simulink model "lr_pwm"  (R2021b)
settings: Solver=ode1  StartTime=0.0  StopTime=3  FixedStep=T_sim  RelTol=1e-3  AbsTol=1e-3
values from neighbouring files (symbols this model uses):
  Ac_s = [-1/(C_s*R_s)    1/C_s ... (first row only)    [lr_pwm_data.m]
  Ao_s = [-1/(C_s*R_s)    1/C_s ... (first row only)    [lr_pwm_data.m]
  Bc_s = [0;1/L_l]    [lr_pwm_data.m]
  Bo_s = [0;1/(L_l)]    [lr_pwm_data.m]
  Cc_s = [1/R_s 0]    [lr_pwm_data.m]
  Co_s = [0 1]    [lr_pwm_data.m]
  Dc_s = zeros(p,m)    [lr_pwm_data.m]
  delta = 0.001    [lr_pwm_data.m]
  deltao = 0.001    [lr_pwm_data.m]
  FR = -diag([1/0.01])    [lr_pwm_data.m]
  L = 200e-3    (= 0.2)    [Parameter_Vergleich.m]
  Lam_inv = inv(Lam)    [lr_pwm_data.m]
  R_l = 4    [lr_pwm_data.m]
  R_s = 0.1    [lr_pwm_data.m]
  rho = 1    [lr_pwm_data.m]
  rhoo = 5    [lr_pwm_data.m]
  SampleTime = 0.001    [lr_pwm_data.m]
  To_inv = eye(n)    [lr_pwm_data.m]
  U_e = 12    [Parameter_Vergleich.m]    (also in lr_pwm_data.m = 12.5)
  xb0_z = ( eye(length(Ab_z)) - Ab_z ) \ Bb_z * u0    [lr_pwm_data.m]
  xc0_s = ( -Ac_s ) * Bc_s .\ u0    [lr_pwm_data.m]
  xc0_z = ( eye(length(Ac_z)) - Ac_z ) \ Bc_z * u0    [lr_pwm_data.m]
  z0 = zeros(1,n)    [lr_pwm_data.m]
undefined symbols (not defined in the file or in its folder): Ab_z, Ac_z, Bb_z, Bc_z, Cb_z, Cc_z, Db_z, Dc_z, DiscIntNeverNeededParam, F, G, Lr, Lrdot, P, S, Sr
libraries: fl_lib x22, nesl_utility x12, simulink x5, ee_lib x1
Description:
  | PWM-Controlled DC Motor
settings Model: DataTypeOverride=Off  MinMaxOverflowLogging=ForceOff  SimulationMode=accelerator  Creator=The MathWorks, Inc.  LastModifiedBy=w.schwamm
settings SolverCC: AutoScaleAbsTol=off  AlgebraicLoopSolver=TrustRegion
settings DataIOCC: LimitDataPoints=on  MaxDataPoints=10000  SaveOutput=off  SaveTime=off  SignalLoggingName=logsout_lr_pwm
settings OptimizationCC: DefaultParameterBehavior=Inlined  EnhancedBackFolding=on  PassReuseOutputArgsAs=Individual arguments  ExpressionDepthLimit=2147483647  ZeroExternalMemoryAtStartup=off  ZeroInternalMemoryAtStartup=off  InitFltsAndDblsToZero=on  OptimizeBlockOrder=speed  DifferentSizesBufferReuse=on  OptimizationCustomize=off  EfficientTunableParamExpr=on
settings DebuggingCC: SignalRangeChecking=error  UnderspecifiedInitializationDetection=Classic  MergeDetectMultiDrivingBlocksExec=none  IntegerOverflowMsg=none  ParameterDowncastMsg=none  ParameterOverflowMsg=none  ParameterPrecisionLossMsg=none  ParameterTunabilityLossMsg=error  FcnCallInpInsideContextMsg=warning  StateNameClashWarn=warning  SFUnexpectedBacktrackingDiag=warning  SFNoUnconditionalDefaultTransitionDiag=warning  SFExecutionAtInitializationDiag=none  SFMachineParentedDataDiag=warning  IntegerSaturationMsg=none  ArithmeticOperatorsInVariantConditions=warning
settings HardwareCC: ProdBitPerPointer=32  ProdBitPerSizeT=32  ProdBitPerPtrDiffT=32  ProdLargestAtomicInteger=Long  ProdLargestAtomicFloat=Double  ProdWordSize=32  ProdHWDeviceType=ARM Compatible->ARM 11
settings ModelReferenceCC: PropagateSignalLabelsOutOfModel=off
settings SFSimCC: SimUseLocalCustomCode=off  MATLABDynamicMemAlloc=off  CustomCodeUndefinedFunction=UseInterfaceOnly
settings RTWCC: Description=Embedded Coder  SystemTargetFile=ert.tlc  TemplateMakefile=ert_default_tmf  RTWUseLocalCustomCode=off
settings CodeAppCC: ForceParamTrailComments=on  IgnoreCustomStorageClasses=off  OperatorAnnotations=on  SimulinkDataObjDesc=on  SFDataObjDesc=on  InsertBlockDesc=on
settings ERTTargetCC: GenerateSampleERTMain=on  InlinedParameterPlacement=NonHierarchical  ERTCustomFileTemplate=example_file_process.tlc
settings ConfigComp: CovMetricSettings=dw  CovSaveCumulativeToWorkspaceVar=on  CovSaveSingleToWorkspaceVar=on  CovExternalEMLEnable=off  CovSFcnEnable=off
settings SimscapeCC: SimscapeLogType=all  SimscapeLogSimulationStatistics=on  SimscapeLogName=simlog_lr_pwm  SimscapeLogDataHistory=10000

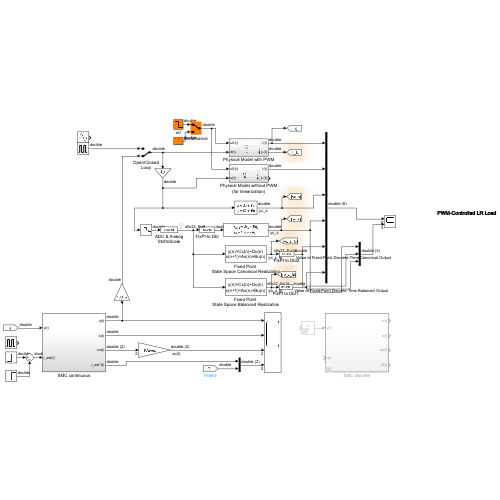
[thumbnail: Simulink's stored preview of the top-level diagram]
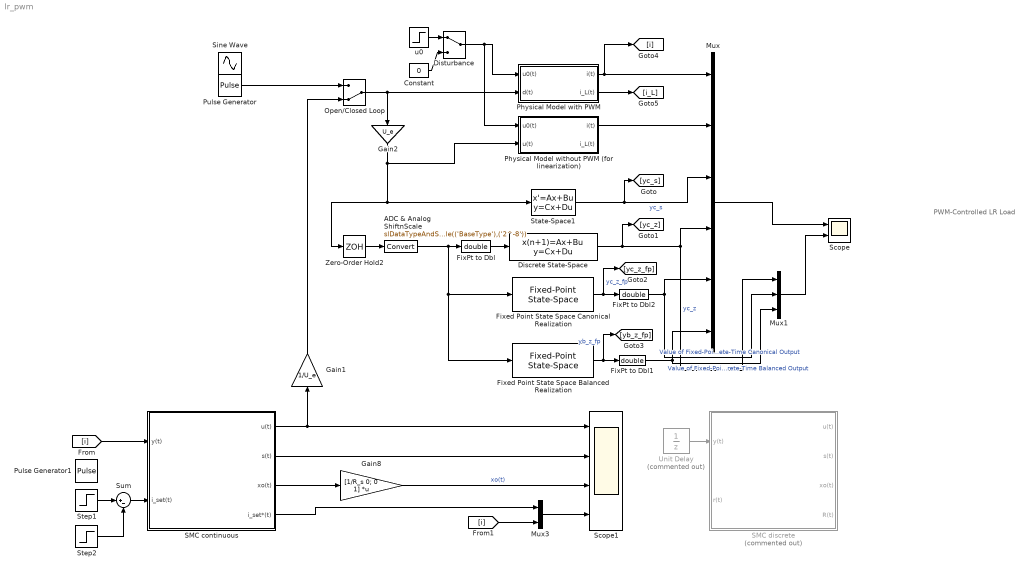
== system lr_pwm ==
  note: PWM-Controlled LR Load
  ADC & Analog ShiftnScale : DataTypeConversion  OutDataTypeStr=slDataTypeAndScale(('BaseType'),('2^-8'))  RndMeth=Nearest  SaturateOnIntegerOverflow=on  LockScale=on
  Constant : Constant  Value=0
  Discrete State-Space : DiscreteStateSpace  A=Ac_z  B=Bc_z  C=Cc_z  D=Dc_z  InitialCondition=xc0_z  SampleTime=SampleTime
  Disturbance : ManualSwitch
  FixPt to Dbl : DataTypeConversion  OutDataTypeStr=double
  FixPt to Dbl1 : DataTypeConversion  OutDataTypeStr=double
  FixPt to Dbl2 : DataTypeConversion  OutDataTypeStr=double
  Fixed Point State Space Balanced Realization : simulink/Additional Math & Discrete/Additional Discrete/Fixed-Point State-Space  A=Ab_z  B=Bb_z  C=Cb_z  D=Db_z  InitialCondition=xb0_z  InternalDataType=BaseType  StateEqScaling=2^(-13)  OutputEqScaling=2^(-15)  DoSatur=off
      settings: SourceProductBaseCode=SL
  Fixed Point State Space Canonical Realization : simulink/Additional Math & Discrete/Additional Discrete/Fixed-Point State-Space  A=Ac_z  B=Bc_z  C=Cc_z  D=Dc_z  InitialCondition=xc0_z  InternalDataType=BaseType  StateEqScaling=2^(-13)  OutputEqScaling=2^(-15)  DoSatur=off
      settings: SourceProductBaseCode=SL
  Gain1 : Gain  Gain=1/U_e
  Gain2 : Gain  Gain=U_e
  Gain8 : Gain  Gain=[1/R_s 0; 0 1]  Multiplication=Matrix(K*u) (u vector)
  Mux : Mux  Inputs=6
  Mux1 : Mux  Inputs=3
  Mux3 : Mux  Inputs=2
  Open/Closed Loop : ManualSwitch  CurrentSetting=0
  Physical Model with PWM : Subsystem
  Physical Model without PWM (for linearization) : Subsystem
  Pulse Generator : DiscretePulseGenerator  PulseType=Time based  Period=0.5  PulseWidth=50
  Pulse Generator1 : DiscretePulseGenerator  PulseType=Time based  Amplitude=1.5  Period=0.5  PulseWidth=50
  SMC continuous : Subsystem  SystemSampleTime=0.001
  SMC discrete : Subsystem  Commented=on  TreatAsAtomicUnit=on  SystemSampleTime=0.001
  Scope : Scope  NumInputPorts=2
  Scope1 : Scope  NumInputPorts=4
  Sine Wave : Sin  Amplitude=0.5  Bias=0.5  Frequency=50  SampleTime=0
  State-Space1 : StateSpace  A=Ac_s  B=Bc_s  C=Cc_s  D=Dc_s  InitialCondition=xc0_s
  Step1 : Step  Time=0.1  After=1.0  SampleTime=0
  Step2 : Step  Time=2  After=0.5  SampleTime=0
  Sum : Sum  Inputs=|+-
  Unit Delay : UnitDelay  Commented=on  SampleTime=-1  HasFrameUpgradeWarning=on
  Zero-Order Hold2 : ZeroOrderHold  SampleTime=SampleTime
  u0 : Step  Time=0.5  After=-3  SampleTime=0
  wires:
  Mux/1 -> Scope/1
  Physical Model without PWM (for linearization)/1(i(t)) -> Mux/2
  State-Space1/1 -> [yc_s], Mux/3  "yc_s"
  Zero-Order Hold2/1 -> ADC & Analog ShiftnScale/1
  ADC & Analog ShiftnScale/1 -> Fixed Point State Space Balanced Realization/1, Fixed Point State Space Canonical Realization/1, FixPt to Dbl/1
  FixPt to Dbl/1 -> Discrete State-Space/1
  Discrete State-Space/1 -> [yc_z], Mux/4, Mux1/1  "yc_z"
  Fixed Point State Space Canonical Realization/1 -> [yc_z_fp], FixPt to Dbl2/1  "yc_z_fp"
  Fixed Point State Space Balanced Realization/1 -> [yb_z_fp], FixPt to Dbl1/1  "yb_z_fp"
  Physical Model with PWM/1(i(t)) -> [i], Mux/1
  FixPt to Dbl2/1 -> Mux1/2, Mux/5  "Value of Fixed-Point Discrete-Time Canonical Output"
  Mux1/1 -> Scope/2
  FixPt to Dbl1/1 -> Mux/6, Mux1/3  "Value of Fixed-Point Discrete-Time Balanced Output"
  Physical Model with PWM/2(i_L(t)) -> [i_L]
  [i] -> Mux3/2
  SMC continuous/1(u(t)) -> Scope1/1, Gain1/1
  Mux3/1 -> Scope1/4
  SMC continuous/2(s(t)) -> Scope1/2
  SMC continuous/3(xo(t)) -> Gain8/1
  Gain8/1 -> Scope1/3  "xo(t)"
  SMC continuous/4(i_set*(t)) -> Mux3/1
  Gain1/1 -> Open/Closed Loop/2
  Step1/1 -> Sum/1
  Sum/1 -> SMC continuous/2(i_set(t))
  Step2/1 -> Sum/2
  u0/1 -> Disturbance/1
  Constant/1 -> Disturbance/2
  Disturbance/1 -> Physical Model without PWM (for linearization)/1(u0(t)), Physical Model with PWM/1(u0(t))
  Open/Closed Loop/1 -> Gain2/1, Physical Model with PWM/2(d(t))
  Pulse Generator/1 -> Open/Closed Loop/1
  Gain2/1 -> Physical Model without PWM (for linearization)/2(u(t)), Zero-Order Hold2/1, State-Space1/1
  Unit Delay/1 -> SMC discrete/1(y(t))
  [i] -> SMC continuous/1(y(t))

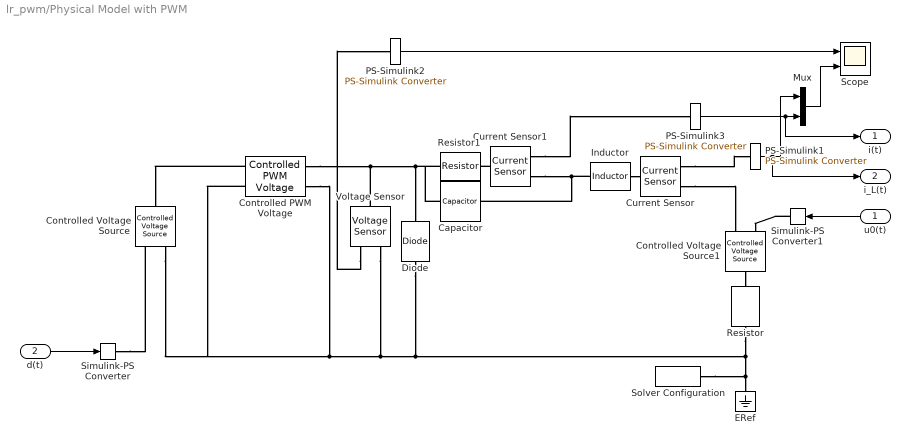
== system lr_pwm/Physical Model with PWM ==
  u0(t) : Inport
  d(t) : Inport  Port=2
  Capacitor : fl_lib/Electrical/Electrical Elements/Capacitor  c=C_s F  r=0 Ohm  g=0 1/Ohm  i_specify=off  i_priority=None  i=0 A  i_nominal_specify=off  i_nominal_unit=A  i_nominal_value=1  v_specify=off  v_priority=None  v=0 V  v_nominal_specify=off  v_nominal_unit=V  v_nominal_value=1  vc_specify=off  vc_priority=High  vc=0 V  vc_nominal_specify=off  vc_nominal_unit=V  vc_nominal_value=1
  Controlled PWM Voltage : ee_lib/Integrated Circuits/Controlled PWM Voltage  F=f_pwm Hz  TD=0 s  pulse_width_offset=0 s  pulse_min=0 s  pwm_or_av=1  event_type=2  sample_time=T_sim s  Vmin=0 V  Vmax=1 V  Vm=U_e V  u_min=0  u_max=1
  Controlled Voltage Source : fl_lib/Electrical/Electrical Sources/Controlled Voltage Source
  Controlled Voltage Source1 : fl_lib/Electrical/Electrical Sources/Controlled Voltage Source
  Current Sensor : fl_lib/Electrical/Electrical Sensors/Current Sensor
  Current Sensor1 : fl_lib/Electrical/Electrical Sensors/Current Sensor
  Diode : fl_lib/Electrical/Electrical Elements/Diode  Vf=0.6 V  Ron=0.3 Ohm  Goff=1e-8 1/Ohm  i_specify=off  i_priority=None  i=0 A  i_nominal_specify=off  i_nominal_unit=A  i_nominal_value=1  v_specify=off  v_priority=None  v=0 V  v_nominal_specify=off  v_nominal_unit=V  v_nominal_value=1
  ERef : fl_lib/Electrical/Electrical Elements/Electrical Reference
  Inductor : fl_lib/Electrical/Electrical Elements/Inductor  l=L_l H  r=0 Ohm  g=0 1/Ohm  i_specify=off  i_priority=None  i=0 A  i_nominal_specify=off  i_nominal_unit=A  i_nominal_value=1  v_specify=off  v_priority=None  v=0 V  v_nominal_specify=off  v_nominal_unit=V  v_nominal_value=1  i_L_specify=off  i_L_priority=High  i_L=0 A  i_L_nominal_specify=off  i_L_nominal_unit=A  i_L_nominal_value=1
  Mux : Mux  Inputs=2
  PS-Simulink1 : nesl_utility/PS-Simulink Converter  PhysicalDomain=network_engine_domain  SubClassName=ps_output  LeftPortType=input  RightPortType=output  PseudoPeriodic=off  Frequencies=[]  Unit=A  AffineConversion=off
      settings: SourceProductBaseCode=PW,SS
  PS-Simulink2 : nesl_utility/PS-Simulink Converter  PhysicalDomain=network_engine_domain  SubClassName=ps_output  LeftPortType=input  RightPortType=output  PseudoPeriodic=off  Frequencies=[]  Unit=V  AffineConversion=off
      settings: SourceProductBaseCode=PW,SS
  PS-Simulink3 : nesl_utility/PS-Simulink Converter  PhysicalDomain=network_engine_domain  SubClassName=ps_output  LeftPortType=input  RightPortType=output  PseudoPeriodic=off  Frequencies=[]  Unit=A  AffineConversion=off
      settings: SourceProductBaseCode=PW,SS
  Resistor : fl_lib/Electrical/Electrical Elements/Resistor  R=R_l Ohm  i_specify=off  i_priority=None  i=0 A  i_nominal_specify=off  i_nominal_unit=A  i_nominal_value=1  v_specify=off  v_priority=None  v=0 V  v_nominal_specify=off  v_nominal_unit=V  v_nominal_value=1
  Resistor1 : fl_lib/Electrical/Electrical Elements/Resistor  R=R_s Ohm  i_specify=off  i_priority=None  i=0 A  i_nominal_specify=off  i_nominal_unit=A  i_nominal_value=1  v_specify=off  v_priority=None  v=0 V  v_nominal_specify=off  v_nominal_unit=V  v_nominal_value=1
  Scope : Scope  NumInputPorts=2
  Simulink-PS Converter : nesl_utility/Simulink-PS Converter  PhysicalDomain=network_engine_domain  SubClassName=ps_input  LeftPortType=input  RightPortType=output  PseudoPeriodic=off  Frequencies=[]  NoiseDistribution=none  NoiseParameters=[]  Unit=1  AffineConversion=off  FilteringAndDerivatives=filter  SimscapeFilterOrder=1  InputFilterTimeConstant=0.001  UdotUserProvided=0
      settings: SourceProductBaseCode=PW,SS
  Simulink-PS Converter1 : nesl_utility/Simulink-PS Converter  PhysicalDomain=network_engine_domain  SubClassName=ps_input  LeftPortType=input  RightPortType=output  PseudoPeriodic=off  Frequencies=[]  NoiseDistribution=none  NoiseParameters=[]  Unit=V  AffineConversion=off  FilteringAndDerivatives=filter  SimscapeFilterOrder=1  InputFilterTimeConstant=0.001  UdotUserProvided=0
      settings: SourceProductBaseCode=PW,SS
  Solver Configuration : nesl_utility/Solver Configuration  PhysicalDomain=network_engine_domain  SubClassName=solver  LeftPortType=input  RightPortType=generic  Tones=[]  Harmonics=[]  SimulateNoise=off  Profile=off  UseLocalSampling=off  EnableSwitchedLinearOptims=on  FrequencyDomain=off  UseCCode=off  RelTol=0.001  AbsTol=1e-06  MinStep=1e-09  ToWorkspace=off  RevertToSquareIcSolve=off  NumHomotopyIterations=100  PhasorMode=off  PhasorModeNumHarmonics=1  DoDC=off  ResidualTolerance=1e-9  UseLocalSolver=off  LocalSolverChoice=NE_BACKWARD_EULER_ADVANCER  LocalSolverSampleTime=5e-6  DoFixedCost=off  MaxNonlinIter=4  MaxModeIter=2  ComputeImpulses=off  ImpulseIterations=2  LinearAlgebra=auto  EquationFormulation=NE_TIME_EF  DelaysMemoryBudget=1024  AutomaticFiltering=off  FilteringTimeConstant=0.001  PartitionStorageMethod=AS_NEEDED  PartitionMemoryBudget=1024  PartitionMethod=FAST
      settings: SourceProductBaseCode=PW,SS
  Voltage Sensor : fl_lib/Electrical/Electrical Sensors/Voltage Sensor
  i(t) : Outport
  i_L(t) : Outport  Port=2
  wires:
  PS-Simulink2/1 -> Scope/1
  d(t)/1 -> Simulink-PS Converter/1
  PS-Simulink3/1 -> i(t)/1, Mux/2
  Mux/1 -> Scope/2
  PS-Simulink1/1 -> i_L(t)/1, Mux/1
  u0(t)/1 -> Simulink-PS Converter1/1
  connections:
  Voltage Sensor/LConn1 -- Capacitor/LConn1 -- Resistor1/LConn1 -- Diode/RConn1 -- Controlled PWM Voltage/RConn1
  Inductor/RConn1 -- Current Sensor/LConn1
  Voltage Sensor/RConn2 -- Controlled PWM Voltage/RConn2 -- Controlled PWM Voltage/LConn2 -- Controlled Voltage Source/RConn2 -- Diode/LConn1 -- Resistor/RConn1 -- Solver Configuration/RConn1 -- ERef/LConn1
  Inductor/LConn1 -- Current Sensor1/RConn2 -- Capacitor/RConn1
  Simulink-PS Converter/RConn1 -- Controlled Voltage Source/RConn1
  Current Sensor1/LConn1 -- Resistor1/RConn1
  Current Sensor1/RConn1 -- PS-Simulink3/LConn1
  Current Sensor/RConn1 -- PS-Simulink1/LConn1
  Voltage Sensor/RConn1 -- PS-Simulink2/LConn1
  Controlled PWM Voltage/LConn1 -- Controlled Voltage Source/LConn1
  Simulink-PS Converter1/RConn1 -- Controlled Voltage Source1/RConn1
  Controlled Voltage Source1/LConn1 -- Resistor/LConn1
  Current Sensor/RConn2 -- Controlled Voltage Source1/RConn2

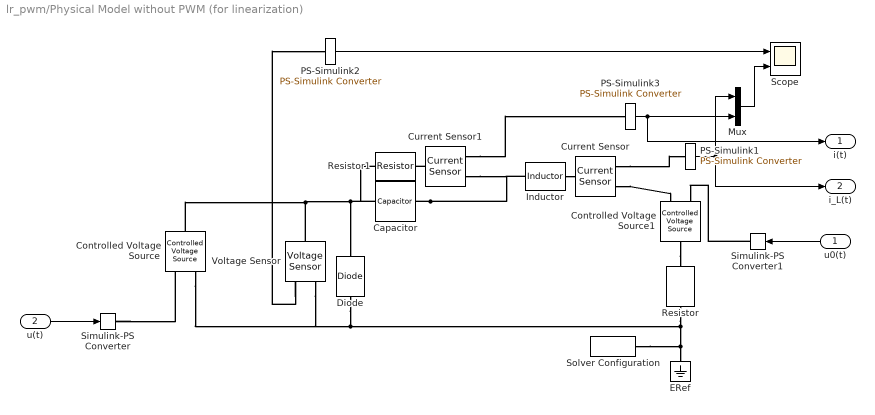
== system lr_pwm/Physical Model without PWM (for linearization) ==
  u0(t) : Inport
  u(t) : Inport  Port=2
  Capacitor : fl_lib/Electrical/Electrical Elements/Capacitor  c=C_s F  r=0 Ohm  g=0 1/Ohm  i_specify=off  i_priority=None  i=0 A  i_nominal_specify=off  i_nominal_unit=A  i_nominal_value=1  v_specify=off  v_priority=None  v=0 V  v_nominal_specify=off  v_nominal_unit=V  v_nominal_value=1  vc_specify=off  vc_priority=High  vc=0 V  vc_nominal_specify=off  vc_nominal_unit=V  vc_nominal_value=1
  Controlled Voltage Source : fl_lib/Electrical/Electrical Sources/Controlled Voltage Source
  Controlled Voltage Source1 : fl_lib/Electrical/Electrical Sources/Controlled Voltage Source
  Current Sensor : fl_lib/Electrical/Electrical Sensors/Current Sensor
  Current Sensor1 : fl_lib/Electrical/Electrical Sensors/Current Sensor
  Diode : fl_lib/Electrical/Electrical Elements/Diode  Vf=0.6 V  Ron=0.3 Ohm  Goff=1e-8 1/Ohm  i_specify=off  i_priority=None  i=0 A  i_nominal_specify=off  i_nominal_unit=A  i_nominal_value=1  v_specify=off  v_priority=None  v=0 V  v_nominal_specify=off  v_nominal_unit=V  v_nominal_value=1
  ERef : fl_lib/Electrical/Electrical Elements/Electrical Reference
  Inductor : fl_lib/Electrical/Electrical Elements/Inductor  l=L_l H  r=0 Ohm  g=0 1/Ohm  i_specify=off  i_priority=None  i=0 A  i_nominal_specify=off  i_nominal_unit=A  i_nominal_value=1  v_specify=off  v_priority=None  v=0 V  v_nominal_specify=off  v_nominal_unit=V  v_nominal_value=1  i_L_specify=off  i_L_priority=High  i_L=0 A  i_L_nominal_specify=off  i_L_nominal_unit=A  i_L_nominal_value=1
  Mux : Mux  Inputs=2
  PS-Simulink1 : nesl_utility/PS-Simulink Converter  PhysicalDomain=network_engine_domain  SubClassName=ps_output  LeftPortType=input  RightPortType=output  PseudoPeriodic=off  Frequencies=[]  Unit=A  AffineConversion=off
      settings: SourceProductBaseCode=PW,SS
  PS-Simulink2 : nesl_utility/PS-Simulink Converter  PhysicalDomain=network_engine_domain  SubClassName=ps_output  LeftPortType=input  RightPortType=output  PseudoPeriodic=off  Frequencies=[]  Unit=V  AffineConversion=off
      settings: SourceProductBaseCode=PW,SS
  PS-Simulink3 : nesl_utility/PS-Simulink Converter  PhysicalDomain=network_engine_domain  SubClassName=ps_output  LeftPortType=input  RightPortType=output  PseudoPeriodic=off  Frequencies=[]  Unit=A  AffineConversion=off
      settings: SourceProductBaseCode=PW,SS
  Resistor : fl_lib/Electrical/Electrical Elements/Resistor  R=R_l Ohm  i_specify=off  i_priority=None  i=0 A  i_nominal_specify=off  i_nominal_unit=A  i_nominal_value=1  v_specify=off  v_priority=None  v=0 V  v_nominal_specify=off  v_nominal_unit=V  v_nominal_value=1
  Resistor1 : fl_lib/Electrical/Electrical Elements/Resistor  R=R_s Ohm  i_specify=off  i_priority=None  i=0 A  i_nominal_specify=off  i_nominal_unit=A  i_nominal_value=1  v_specify=off  v_priority=None  v=0 V  v_nominal_specify=off  v_nominal_unit=V  v_nominal_value=1
  Scope : Scope  NumInputPorts=2
  Simulink-PS Converter : nesl_utility/Simulink-PS Converter  PhysicalDomain=network_engine_domain  SubClassName=ps_input  LeftPortType=input  RightPortType=output  PseudoPeriodic=off  Frequencies=[]  NoiseDistribution=none  NoiseParameters=[]  Unit=1  AffineConversion=off  FilteringAndDerivatives=provide  SimscapeFilterOrder=1  InputFilterTimeConstant=0.001  UdotUserProvided=0
      settings: SourceProductBaseCode=PW,SS
  Simulink-PS Converter1 : nesl_utility/Simulink-PS Converter  PhysicalDomain=network_engine_domain  SubClassName=ps_input  LeftPortType=input  RightPortType=output  PseudoPeriodic=off  Frequencies=[]  NoiseDistribution=none  NoiseParameters=[]  Unit=V  AffineConversion=off  FilteringAndDerivatives=filter  SimscapeFilterOrder=1  InputFilterTimeConstant=0.001  UdotUserProvided=0
      settings: SourceProductBaseCode=PW,SS
  Solver Configuration : nesl_utility/Solver Configuration  PhysicalDomain=network_engine_domain  SubClassName=solver  LeftPortType=input  RightPortType=generic  Tones=[]  Harmonics=[]  SimulateNoise=off  Profile=off  UseLocalSampling=off  EnableSwitchedLinearOptims=on  FrequencyDomain=off  UseCCode=off  RelTol=0.001  AbsTol=1e-06  MinStep=1e-09  ToWorkspace=off  RevertToSquareIcSolve=off  NumHomotopyIterations=100  PhasorMode=off  PhasorModeNumHarmonics=1  DoDC=off  ResidualTolerance=1e-9  UseLocalSolver=off  LocalSolverChoice=NE_BACKWARD_EULER_ADVANCER  LocalSolverSampleTime=5e-6  DoFixedCost=off  MaxNonlinIter=4  MaxModeIter=2  ComputeImpulses=off  ImpulseIterations=2  LinearAlgebra=auto  EquationFormulation=NE_TIME_EF  DelaysMemoryBudget=1024  AutomaticFiltering=off  FilteringTimeConstant=0.001  PartitionStorageMethod=AS_NEEDED  PartitionMemoryBudget=1024  PartitionMethod=FAST
      settings: SourceProductBaseCode=PW,SS
  Voltage Sensor : fl_lib/Electrical/Electrical Sensors/Voltage Sensor
  i(t) : Outport
  i_L(t) : Outport  Port=2
  wires:
  PS-Simulink1/1 -> Mux/1, i_L(t)/1
  Mux/1 -> Scope/2
  PS-Simulink3/1 -> Mux/2, i(t)/1
  u(t)/1 -> Simulink-PS Converter/1
  PS-Simulink2/1 -> Scope/1
  u0(t)/1 -> Simulink-PS Converter1/1
  connections:
  Voltage Sensor/RConn1 -- PS-Simulink2/LConn1
  Current Sensor/RConn1 -- PS-Simulink1/LConn1
  Current Sensor1/RConn1 -- PS-Simulink3/LConn1
  Current Sensor1/LConn1 -- Resistor1/RConn1
  Capacitor/RConn1 -- Current Sensor1/RConn2 -- Inductor/LConn1
  Voltage Sensor/RConn2 -- Controlled Voltage Source/RConn2 -- ERef/LConn1 -- Solver Configuration/RConn1 -- Resistor/RConn1 -- Diode/LConn1
  Inductor/RConn1 -- Current Sensor/LConn1
  Controlled Voltage Source/LConn1 -- Voltage Sensor/LConn1 -- Diode/RConn1 -- Resistor1/LConn1 -- Capacitor/LConn1
  Simulink-PS Converter1/RConn1 -- Controlled Voltage Source1/RConn1
  Controlled Voltage Source1/LConn1 -- Resistor/LConn1
  Current Sensor/RConn2 -- Controlled Voltage Source1/RConn2
  Simulink-PS Converter/RConn1 -- Controlled Voltage Source/RConn1

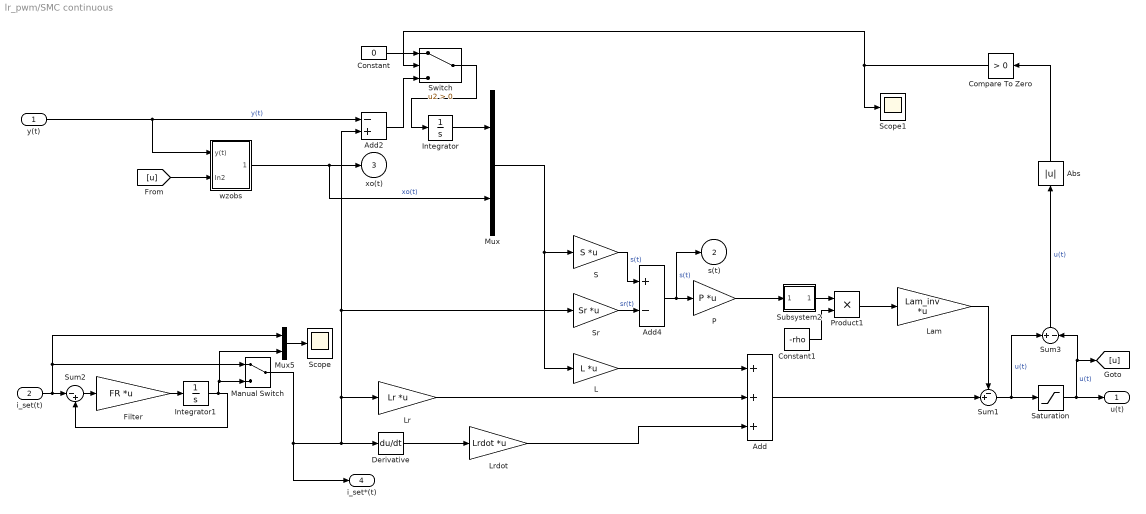
== system lr_pwm/SMC continuous ==
  y(t) : Inport
  i_set(t) : Inport  Port=2
  Abs : Abs
  Add : Sum  Inputs=+++
  Add2 : Sum  Inputs=-+
  Add4 : Sum  Inputs=+-
  Compare To Zero : simulink/Logic and Bit Operations/Compare To Zero  relop=>  OutDataTypeStr=boolean
  Constant : Constant  Value=0
  Constant1 : Constant  Value=-rho  SampleTime=-1
  Derivative : Derivative
  Filter : Gain  Gain=FR  Multiplication=Matrix(K*u) (u vector)
  Integrator : Integrator
  Integrator1 : Integrator
  L : Gain  Gain=L  Multiplication=Matrix(K*u) (u vector)
  Lam : Gain  Gain=Lam_inv  Multiplication=Matrix(K*u) (u vector)
  Lr : Gain  Gain=Lr  Multiplication=Matrix(K*u) (u vector)
  Lrdot : Gain  Gain=Lrdot  Multiplication=Matrix(K*u) (u vector)
  Manual Switch : ManualSwitch
  Mux : Mux  Inputs=2
  Mux5 : Mux  Inputs=2
  P : Gain  Gain=P  Multiplication=Matrix(K*u) (u vector)
  Product1 : Product
  S : Gain  Gain=S  Multiplication=Matrix(K*u) (u vector)
  Saturation : Saturate  UpperLimit=U_e  LowerLimit=0
  Scope : Scope
  Scope1 : Scope
  Sr : Gain  Gain=Sr  Multiplication=Matrix(K*u) (u vector)
  Subsystem2 : Subsystem  mask{delta=delta}
      mask prompts: delta "Unit vector delta:"
      mask Display: disp('UnV')
  Sum1 : Sum  Inputs=-+|
  Sum2 : Sum  Inputs=|-+
  Sum3 : Sum  Inputs=+-
  Switch : Switch  Criteria=u2 > Threshold
  wzobs : Subsystem
  u(t) : Outport  VectorParamsAs1DForOutWhenUnconnected=off
  s(t) : Outport  Port=2
  xo(t) : Outport  Port=3
  i_set*(t) : Outport  Port=4  VectorParamsAs1DForOutWhenUnconnected=off
  wires:
  Constant1/1 -> Product1/2
  Subsystem2/1(Out1) -> Product1/1
  Lrdot/1 -> Add/3
  Lr/1 -> Add/2
  Sr/1 -> Add4/2  "sr(t)"
  Switch/1 -> Integrator/1
  Integrator1/1 -> Manual Switch/2, Mux5/2, Sum2/2
  Constant/1 -> Switch/1
  Add2/1 -> Switch/3
  Compare To Zero/1 -> Scope1/1, Switch/2
  Abs/1 -> Compare To Zero/1
  Sum3/1 -> Abs/1  "u(t)"
  Saturation/1 -> u(t)/1, [u], Sum3/2  "u(t)"
  Mux5/1 -> Scope/1
  Filter/1 -> Integrator1/1
  Sum2/1 -> Filter/1
  i_set(t)/1 -> Sum2/1, Manual Switch/1, Mux5/1
  Add/1 -> Sum1/2
  P/1 -> Subsystem2/1(In1)
  Sum1/1 -> Saturation/1, Sum3/1  "u(t)"
  Add4/1 -> s(t)/1, P/1  "s(t)"
  Integrator/1 -> Mux/1
  L/1 -> Add/1
  Mux/1 -> L/1, S/1
  Manual Switch/1 -> Derivative/1, Sr/1, Add2/2, Lr/1, i_set*(t)/1
  Lam/1 -> Sum1/1
  S/1 -> Add4/1  "s(t)"
  Derivative/1 -> Lrdot/1
  [u] -> wzobs/2(In2)
  wzobs/1(xo(t)) -> xo(t)/1, Mux/2  "xo(t)"
  y(t)/1 -> wzobs/1(y(t)), Add2/1  "y(t)"
  Product1/1 -> Lam/1

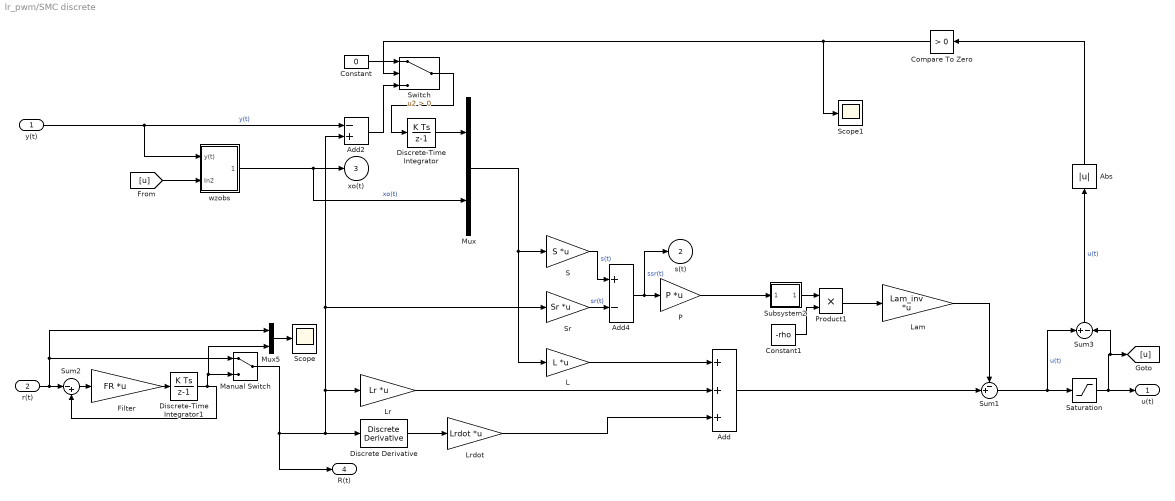
== system lr_pwm/SMC discrete ==
  y(t) : Inport
  r(t) : Inport  Port=2
  Abs : Abs
  Add : Sum  Inputs=+++
  Add2 : Sum  Inputs=-+
  Add4 : Sum  Inputs=+-
  Compare To Zero : simulink/Logic and Bit Operations/Compare To Zero  relop=>  OutDataTypeStr=boolean
  Constant : Constant  Value=0
  Constant1 : Constant  Value=-rho  SampleTime=-1
  Discrete Derivative : simulink/Discrete/Discrete Derivative  gainval=1.0  ICPrevScaledInput=0.0  OutMin=[]  OutMax=[]  OutDataType=fixdt(1, 16)  OutScaling=2^-10  DoSatur=off
  Discrete-Time Integrator : DiscreteIntegrator  SampleTime=-1  ICPrevOutput=DiscIntNeverNeededParam  ICPrevScaledInput=DiscIntNeverNeededParam
  Discrete-Time Integrator1 : DiscreteIntegrator  SampleTime=-1  ICPrevOutput=DiscIntNeverNeededParam  ICPrevScaledInput=DiscIntNeverNeededParam
  Filter : Gain  Gain=FR  Multiplication=Matrix(K*u) (u vector)
  L : Gain  Gain=L  Multiplication=Matrix(K*u) (u vector)
  Lam : Gain  Gain=Lam_inv  Multiplication=Matrix(K*u) (u vector)
  Lr : Gain  Gain=Lr  Multiplication=Matrix(K*u) (u vector)
  Lrdot : Gain  Gain=Lrdot  Multiplication=Matrix(K*u) (u vector)
  Manual Switch : ManualSwitch
  Mux : Mux  Inputs=2
  Mux5 : Mux  Inputs=2
  P : Gain  Gain=P  Multiplication=Matrix(K*u) (u vector)
  Product1 : Product
  S : Gain  Gain=S  Multiplication=Matrix(K*u) (u vector)
  Saturation : Saturate  UpperLimit=U_e  LowerLimit=0
  Scope : Scope
  Scope1 : Scope
  Sr : Gain  Gain=Sr  Multiplication=Matrix(K*u) (u vector)
  Subsystem2 : Subsystem  mask{delta=delta}
      mask prompts: delta "Unit vector delta:"
      mask Display: disp('UnV')
  Sum1 : Sum  Inputs=-+|
  Sum2 : Sum  Inputs=|-+
  Sum3 : Sum  Inputs=+-
  Switch : Switch  Criteria=u2 > Threshold
  wzobs : Subsystem
  u(t) : Outport  VectorParamsAs1DForOutWhenUnconnected=off
  s(t) : Outport  Port=2
  xo(t) : Outport  Port=3
  R(t) : Outport  Port=4  VectorParamsAs1DForOutWhenUnconnected=off
  wires:
  y(t)/1 -> Add2/1, wzobs/1(y(t))  "y(t)"
  wzobs/1(xo(t)) -> Mux/2, xo(t)/1  "xo(t)"
  [u] -> wzobs/2(In2)
  Discrete Derivative/1 -> Lrdot/1
  S/1 -> Add4/1  "s(t)"
  Lam/1 -> Sum1/1
  Manual Switch/1 -> R(t)/1, Lr/1, Add2/2, Sr/1, Discrete Derivative/1
  Mux/1 -> S/1, L/1
  L/1 -> Add/1
  Discrete-Time Integrator/1 -> Mux/1
  Add4/1 -> P/1, s(t)/1  "ssr(t)"
  Sum1/1 -> Sum3/1, Saturation/1  "u(t)"
  P/1 -> Subsystem2/1(In1)
  Add/1 -> Sum1/2
  r(t)/1 -> Mux5/1, Manual Switch/1, Sum2/1
  Sum2/1 -> Filter/1
  Filter/1 -> Discrete-Time Integrator1/1
  Mux5/1 -> Scope/1
  Saturation/1 -> Sum3/2, [u], u(t)/1
  Sum3/1 -> Abs/1  "u(t)"
  Abs/1 -> Compare To Zero/1
  Compare To Zero/1 -> Scope1/1, Switch/2
  Add2/1 -> Switch/3
  Constant/1 -> Switch/1
  Discrete-Time Integrator1/1 -> Sum2/2, Mux5/2, Manual Switch/2
  Switch/1 -> Discrete-Time Integrator/1
  Sr/1 -> Add4/2  "sr(t)"
  Lr/1 -> Add/2
  Lrdot/1 -> Add/3
  Subsystem2/1(Out1) -> Product1/1
  Constant1/1 -> Product1/2
  Product1/1 -> Lam/1

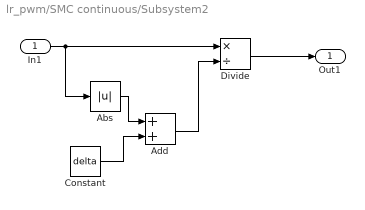
== system lr_pwm/SMC continuous/Subsystem2 ==
  In1 : Inport
  Abs : Abs  ZeroCross=off
  Add : Sum
  Constant : Constant  Value=delta  SampleTime=-1
  Divide : Product  Inputs=*/
  Out1 : Outport
  wires:
  Constant/1 -> Add/2
  Add/1 -> Divide/2
  Abs/1 -> Add/1
  Divide/1 -> Out1/1
  In1/1 -> Divide/1, Abs/1

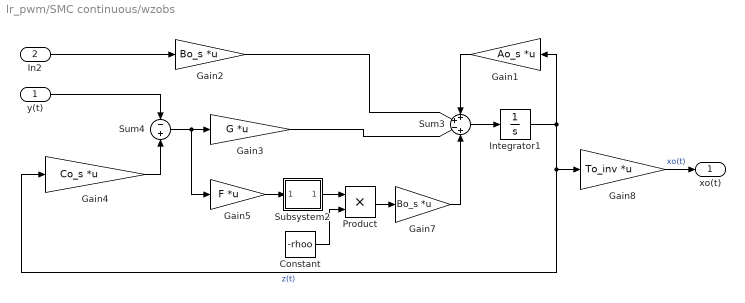
== system lr_pwm/SMC continuous/wzobs ==
  y(t) : Inport
  In2 : Inport  Port=2
  Constant : Constant  Value=-rhoo  SampleTime=-1
  Gain1 : Gain  Gain=Ao_s  Multiplication=Matrix(K*u) (u vector)
  Gain2 : Gain  Gain=Bo_s  Multiplication=Matrix(K*u) (u vector)
  Gain3 : Gain  Gain=G  Multiplication=Matrix(K*u) (u vector)
  Gain4 : Gain  Gain=Co_s  Multiplication=Matrix(K*u) (u vector)
  Gain5 : Gain  Gain=F  Multiplication=Matrix(K*u) (u vector)
  Gain7 : Gain  Gain=Bo_s  Multiplication=Matrix(K*u) (u vector)
  Gain8 : Gain  Gain=To_inv  Multiplication=Matrix(K*u) (u vector)
  Integrator1 : Integrator  InitialCondition=z0
  Product : Product
  Subsystem2 : Subsystem  mask{delta=deltao}
      mask prompts: delta "Unit vector delta:"
      mask Display: disp('UnV')
  Sum3 : Sum  Inputs=++-+
  Sum4 : Sum  Inputs=-+
  xo(t) : Outport
  wires:
  Sum4/1 -> Gain5/1, Gain3/1
  Integrator1/1 -> Gain4/1, Gain8/1, Gain1/1  "z(t)"
  Gain4/1 -> Sum4/2
  Gain2/1 -> Sum3/2
  Product/1 -> Gain7/1
  Gain5/1 -> Subsystem2/1(In1)
  Subsystem2/1(Out1) -> Product/1
  Gain7/1 -> Sum3/4
  Gain3/1 -> Sum3/3
  Gain1/1 -> Sum3/1
  Sum3/1 -> Integrator1/1
  In2/1 -> Gain2/1
  y(t)/1 -> Sum4/1
  Constant/1 -> Product/2
  Gain8/1 -> xo(t)/1  "xo(t)"

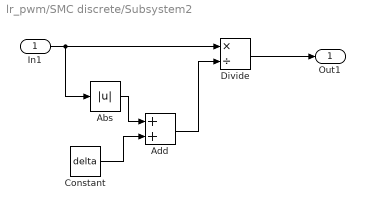
== system lr_pwm/SMC discrete/Subsystem2 ==
  In1 : Inport
  Abs : Abs  ZeroCross=off
  Add : Sum
  Constant : Constant  Value=delta  SampleTime=-1
  Divide : Product  Inputs=*/
  Out1 : Outport
  wires:
  In1/1 -> Abs/1, Divide/1
  Divide/1 -> Out1/1
  Abs/1 -> Add/1
  Add/1 -> Divide/2
  Constant/1 -> Add/2

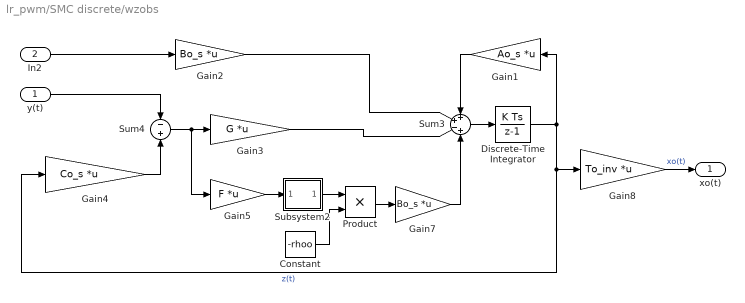
== system lr_pwm/SMC discrete/wzobs ==
  y(t) : Inport
  In2 : Inport  Port=2
  Constant : Constant  Value=-rhoo  SampleTime=-1
  Discrete-Time Integrator : DiscreteIntegrator  SampleTime=-1  ICPrevOutput=DiscIntNeverNeededParam  ICPrevScaledInput=DiscIntNeverNeededParam
  Gain1 : Gain  Gain=Ao_s  Multiplication=Matrix(K*u) (u vector)
  Gain2 : Gain  Gain=Bo_s  Multiplication=Matrix(K*u) (u vector)
  Gain3 : Gain  Gain=G  Multiplication=Matrix(K*u) (u vector)
  Gain4 : Gain  Gain=Co_s  Multiplication=Matrix(K*u) (u vector)
  Gain5 : Gain  Gain=F  Multiplication=Matrix(K*u) (u vector)
  Gain7 : Gain  Gain=Bo_s  Multiplication=Matrix(K*u) (u vector)
  Gain8 : Gain  Gain=To_inv  Multiplication=Matrix(K*u) (u vector)
  Product : Product
  Subsystem2 : Subsystem  mask{delta=deltao}
      mask prompts: delta "Unit vector delta:"
      mask Display: disp('UnV')
  Sum3 : Sum  Inputs=++-+
  Sum4 : Sum  Inputs=-+
  xo(t) : Outport
  wires:
  Gain8/1 -> xo(t)/1  "xo(t)"
  Constant/1 -> Product/2
  y(t)/1 -> Sum4/1
  In2/1 -> Gain2/1
  Sum3/1 -> Discrete-Time Integrator/1
  Gain1/1 -> Sum3/1
  Gain3/1 -> Sum3/3
  Gain7/1 -> Sum3/4
  Subsystem2/1(Out1) -> Product/1
  Gain5/1 -> Subsystem2/1(In1)
  Product/1 -> Gain7/1
  Gain2/1 -> Sum3/2
  Gain4/1 -> Sum4/2
  Discrete-Time Integrator/1 -> Gain1/1, Gain8/1, Gain4/1  "z(t)"
  Sum4/1 -> Gain3/1, Gain5/1

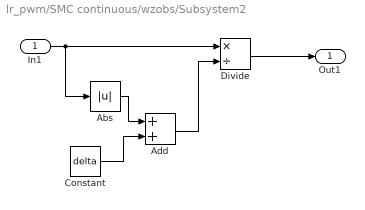
== system lr_pwm/SMC continuous/wzobs/Subsystem2 ==
  In1 : Inport
  Abs : Abs  ZeroCross=off
  Add : Sum
  Constant : Constant  Value=delta  SampleTime=-1
  Divide : Product  Inputs=*/
  Out1 : Outport
  wires:
  Constant/1 -> Add/2
  Add/1 -> Divide/2
  Abs/1 -> Add/1
  Divide/1 -> Out1/1
  In1/1 -> Divide/1, Abs/1

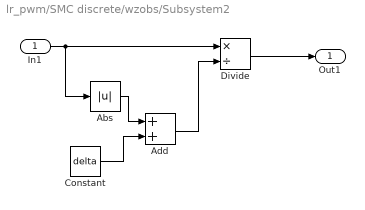
== system lr_pwm/SMC discrete/wzobs/Subsystem2 ==
  In1 : Inport
  Abs : Abs  ZeroCross=off
  Add : Sum
  Constant : Constant  Value=delta  SampleTime=-1
  Divide : Product  Inputs=*/
  Out1 : Outport
  wires:
  In1/1 -> Abs/1, Divide/1
  Divide/1 -> Out1/1
  Abs/1 -> Add/1
  Add/1 -> Divide/2
  Constant/1 -> Add/2
